simulink model "rx2"  (R2022b)
settings: Solver=FixedStepDiscrete  StartTime=0.0  StopTime=3.3E6  FixedStep=1  RelTol=1e-3  EnableMultiTasking=on
model workspace (MAT data in the model file):
  mwTaskManagerKernelLatency = 0
undefined symbols (not defined in the file or in its folder): Add, jsin, magnitude, rom_pilot_conj_tt, Shift
libraries: hdlsllib x3231, whdlutilities x525, simulink x260, whdlmod x112, whdledac x26, dsphdlmathfun2 x24, commchan3 x1
(part 1 of 59)
settings Model: SimulationMode=accelerator  Creator=admin  LastModifiedBy=yangyifei
settings SolverCC: PositivePriorityOrder=on
settings DataIOCC: ExternalInput=data_rx_tt,start_rx_tt,end_rx_tt,valid_rx_tt  LoadExternalInput=on
settings OptimizationCC: DefaultParameterBehavior=Inlined  EnhancedBackFolding=on  PassReuseOutputArgsAs=Individual arguments  ZeroExternalMemoryAtStartup=off  ZeroInternalMemoryAtStartup=off  InitFltsAndDblsToZero=on  MaxStackSize=64  AccelVerboseBuild=on  OptimizeBlockOrder=speed  DifferentSizesBufferReuse=on  OptimizationCustomize=off  EfficientTunableParamExpr=on
settings DebuggingCC: MultiTaskDSMMsg=warning  ParameterTunabilityLossMsg=error
settings HardwareCC: ProdBitPerPointer=32  ProdBitPerSizeT=32  ProdBitPerPtrDiffT=32  ProdLargestAtomicInteger=Long  ProdLargestAtomicFloat=Double  ProdWordSize=32  ProdLongLongMode=on  ProdHWDeviceType=ARM Compatible->ARM Cortex  TargetLongLongMode=on  HardwareBoardFeatureSet=SoCBlockset
settings ModelReferenceCC: EnableRefExpFcnMdlSchedulingChecks=on  ModelReferenceNumInstancesAllowed=Single
settings SFSimCC: MATLABDynamicMemAlloc=off  SimDLAutoTuning=off
settings RTWCC: Description=Embedded Coder  SystemTargetFile=ert.tlc  GenCodeOnly=on  TemplateMakefile=ert_default_tmf  Toolchain=LCC-win64 v2.4.1 | gmake (64-bit Windows)
settings CodeAppCC: ForceParamTrailComments=on  IgnoreCustomStorageClasses=off  OperatorAnnotations=on  SimulinkDataObjDesc=on  SFDataObjDesc=on  InsertBlockDesc=on
settings ERTTargetCC: TargetLangStandard=C99 (ISO)  InlinedParameterPlacement=NonHierarchical  RootIOFormat=Structure reference  ERTCustomFileTemplate=example_file_process.tlc

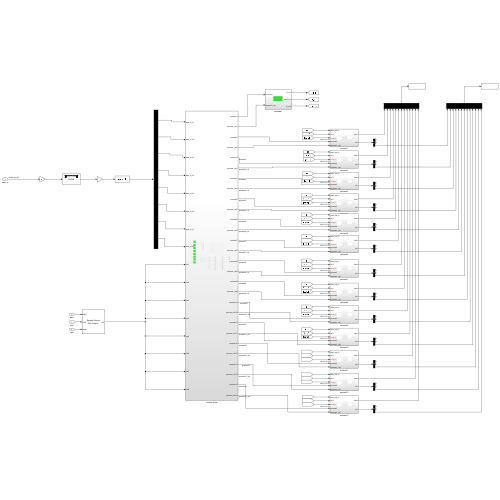
[thumbnail: Simulink's stored preview of the top-level diagram]
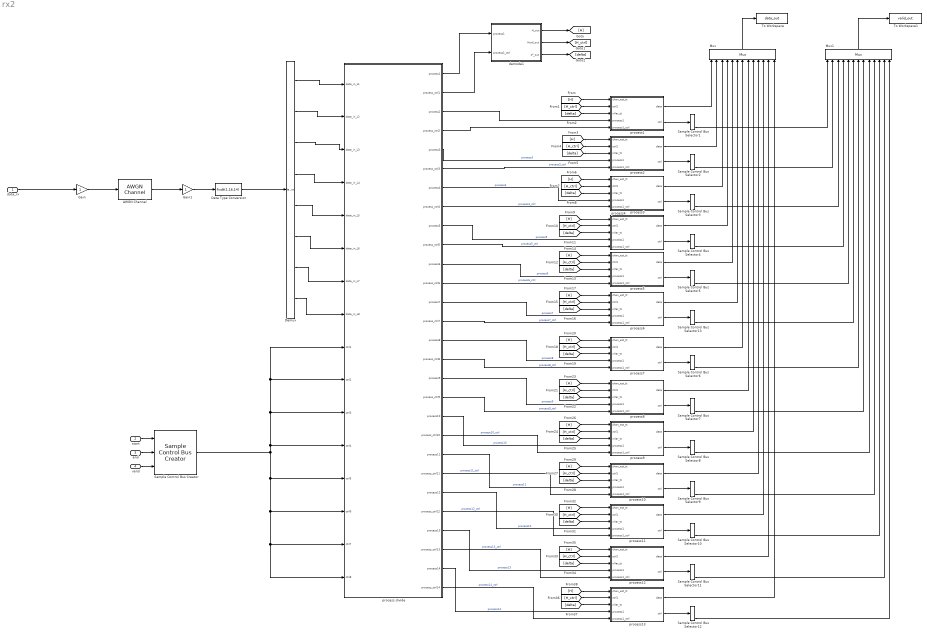
== system rx2 ==
  data_rx : Inport  OutDataTypeStr=double  PortDimensions=8
      settings: SignalType=complex
  start : Inport  Port=2
  end : Inport  Port=3
  valid : Inport  Port=4
  AWGN Channel : commchan3/AWGN Channel  InputProcessing=Columns as channels (frame based)  seed=67  noiseMode="Signal to noise ratio  (SNR)"  EbNodB=10  EsNodB=10  SNRdB=snr  bitsPerSym=1  Ps=1  Tsym=1  variance=1
  Data Type Conversion : DataTypeConversion  OutDataTypeStr=fixdt(1,16,14)  SaturateOnIntegerOverflow=off  RndMeth=Floor
  Demux : Demux  Outputs=8
  Gain : Gain
  Gain1 : Gain
  Mux : Mux  Inputs=13
  Mux1 : Mux  Inputs=13
  Sample Control Bus Creator : whdlutilities/Sample Control Bus Creator
  Sample Control Bus Selector{1..13} (13 alike) : whdlutilities/Sample Control Bus Selector  OutputSignals=start,end,valid
  To Workspace : ToWorkspace  VariableName=data_out  SaveFormat=Timeseries  SampleTime=-1
  To Workspace1 : ToWorkspace  VariableName=valid_out  SaveFormat=Timeseries  SampleTime=-1
  demode1 : Subsystem
  process divide : Subsystem
  process1 : Subsystem
  process10 : Subsystem
  process11 : Subsystem
  process12 : Subsystem
  process13 : Subsystem
  process2 : Subsystem
  process3 : Subsystem
  process4 : Subsystem
  process5 : Subsystem
  process6 : Subsystem
  process7 : Subsystem
  process8 : Subsystem
  process9 : Subsystem
  wires:
  process divide/20(process_ctrl10) -> process9/5(process1_ctrl)  "process10_ctrl"
  Demux/3 -> process divide/3(data_in_L3)
  process divide/13(process7) -> process6/4(process1)  "process7"
  process divide/18(process_ctrl9) -> process8/5(process1_ctrl)  "process9_ctrl"
  Demux/1 -> process divide/1(data_in_L1)
  process divide/14(process_ctrl7) -> process6/5(process1_ctrl)  "process7_ctrl"
  process divide/15(process8) -> process7/4(process1)  "process8"
  Demux/7 -> process divide/7(data_in_L7)
  process divide/8(process_ctrl4) -> process3/5(process1_ctrl)  "process4_ctrl"
  process divide/11(process6) -> process5/4(process1)  "process6"
  process divide/5(process3) -> process2/4(process1)  "process3"
  process divide/7(process4) -> process3/4(process1)  "process4"
  process divide/10(process_ctrl5) -> process4/5(process1_ctrl)  "process5_ctrl"
  process divide/9(process5) -> process4/4(process1)  "process5"
  process divide/3(process2) -> process1/4(process1)
  process divide/6(process_ctrl3) -> process2/5(process1_ctrl)  "process3_ctrl"
  [delta] -> process10/3(nVar_tt)
  [H] -> process9/1(chan_est_tt)
  [delta] -> process13/3(nVar_tt)
  [H_ctrl] -> process2/2(ctrl1)
  [delta] -> process11/3(nVar_tt)
  [H_ctrl] -> process11/2(ctrl1)
  process divide/26(process_ctrl13) -> process12/5(process1_ctrl)  "process13_ctrl"
  [H] -> process12/1(chan_est_tt)
  [H_ctrl] -> process10/2(ctrl1)
  process divide/27(process14) -> process13/4(process1)  "process14"
  process divide/17(process9) -> process8/4(process1)  "process9"
  [delta] -> process6/3(nVar_tt)
  process divide/1(process1) -> demode1/1(process1)
  [H] -> process11/1(chan_est_tt)
  [delta] -> process7/3(nVar_tt)
  demode1/2(Hcrtl_out) -> [H_ctrl]
  [H_ctrl] -> process8/2(ctrl1)
  process divide/19(process10) -> process9/4(process1)  "process10"
  Demux/6 -> process divide/6(data_in_L6)
  [H] -> process7/1(chan_est_tt)
  [delta] -> process5/3(nVar_tt)
  [H] -> process13/1(chan_est_tt)
  process divide/23(process12) -> process11/4(process1)  "process12"
  demode1/3(σ²_out) -> [delta]
  [H] -> process6/1(chan_est_tt)
  [H_ctrl] -> process4/2(ctrl1)
  [delta] -> process12/3(nVar_tt)
  [H] -> process8/1(chan_est_tt)
  [H_ctrl] -> process7/2(ctrl1)
  [delta] -> process2/3(nVar_tt)
  [H_ctrl] -> process6/2(ctrl1)
  process divide/22(process_ctrl11) -> process10/5(process1_ctrl)  "process11_ctrl"
  [delta] -> process4/3(nVar_tt)
  [delta] -> process3/3(nVar_tt)
  Demux/2 -> process divide/2("data_in_L2 ")
  [delta] -> process9/3(nVar_tt)
  [delta] -> process8/3(nVar_tt)
  [H_ctrl] -> process3/2(ctrl1)
  process divide/25(process13) -> process12/4(process1)  "process13"
  [H] -> process5/1(chan_est_tt)
  [H] -> process4/1(chan_est_tt)
  [H] -> process10/1(chan_est_tt)
  [H_ctrl] -> process9/2(ctrl1)
  process divide/21(process11) -> process10/4(process1)  "process11"
  process divide/28(process_ctrl14) -> process13/5(process1_ctrl)  "process14_ctrl"
  Demux/5 -> process divide/5(data_in_L5)
  Demux/8 -> process divide/8(data_in_L8)
  [H_ctrl] -> process12/2(ctrl1)
  [delta] -> process1/3(nVar_tt)
  [H_ctrl] -> process13/2(ctrl1)
  [H] -> process1/1(chan_est_tt)
  [H_ctrl] -> process1/2(ctrl1)
  [H] -> process2/1(chan_est_tt)
  [H_ctrl] -> process5/2(ctrl1)
  process divide/16(process_ctrl8) -> process7/5(process1_ctrl)  "process8_ctrl"
  process divide/24(process_ctrl12) -> process11/5(process1_ctrl)  "process12_ctrl"
  process divide/2(process_ctrl1) -> demode1/2(process1_ctrl)
  process divide/12(process_ctrl6) -> process5/5(process1_ctrl)  "process6_ctrl"
  process divide/4(process_ctrl2) -> process1/5(process1_ctrl)
  demode1/1(H_out) -> [H]
  Demux/4 -> process divide/4(data_in_L4)
  [H] -> process3/1(chan_est_tt)
  start/1 -> Sample Control Bus Creator/1
  end/1 -> Sample Control Bus Creator/2
  valid/1 -> Sample Control Bus Creator/3
  Sample Control Bus Creator/1 -> process divide/16(ctrl8), process divide/15(ctrl7), process divide/14(ctrl6), process divide/13(ctrl5), process divide/12(ctrl4), process divide/11(ctrl3), process divide/10(ctrl2), process divide/9(ctrl1)
  process1/1(data) -> Mux/1
  process2/1(data) -> Mux/2
  process3/1(data) -> Mux/3
  process4/1(data) -> Mux/4
  process5/1(data) -> Mux/5
  process6/1(data) -> Mux/6
  process7/1(data) -> Mux/7
  process8/1(data) -> Mux/8
  process9/1(data) -> Mux/9
  process10/1(data) -> Mux/10
  process11/1(data) -> Mux/11
  process13/1(data) -> Mux/13
  process12/1(data) -> Mux/12
  Mux/1 -> To Workspace/1
  process1/2(ctrl) -> Sample Control Bus Selector1/1
  process2/2(ctrl) -> Sample Control Bus Selector2/1
  process3/2(ctrl) -> Sample Control Bus Selector3/1
  process4/2(ctrl) -> Sample Control Bus Selector4/1
  process5/2(ctrl) -> Sample Control Bus Selector5/1
  process7/2(ctrl) -> Sample Control Bus Selector6/1
  process8/2(ctrl) -> Sample Control Bus Selector7/1
  process9/2(ctrl) -> Sample Control Bus Selector8/1
  process10/2(ctrl) -> Sample Control Bus Selector9/1
  process11/2(ctrl) -> Sample Control Bus Selector10/1
  process12/2(ctrl) -> Sample Control Bus Selector11/1
  process13/2(ctrl) -> Sample Control Bus Selector12/1
  process6/2(ctrl) -> Sample Control Bus Selector13/1
  Mux1/1 -> To Workspace1/1
  Sample Control Bus Selector1/3 -> Mux1/1
  Sample Control Bus Selector2/3 -> Mux1/2
  Sample Control Bus Selector3/3 -> Mux1/3
  Sample Control Bus Selector4/3 -> Mux1/4
  Sample Control Bus Selector5/3 -> Mux1/5
  Sample Control Bus Selector13/3 -> Mux1/6
  Sample Control Bus Selector6/3 -> Mux1/7
  Sample Control Bus Selector7/3 -> Mux1/8
  Sample Control Bus Selector8/3 -> Mux1/9
  Sample Control Bus Selector9/3 -> Mux1/10
  Sample Control Bus Selector10/3 -> Mux1/11
  Sample Control Bus Selector11/3 -> Mux1/12
  Sample Control Bus Selector12/3 -> Mux1/13
  AWGN Channel/1 -> Gain1/1
  Gain/1 -> AWGN Channel/1
  Gain1/1 -> Data Type Conversion/1
  Data Type Conversion/1 -> Demux/1
  data_rx/1 -> Gain/1

== system rx2/demode1 ==
  process1 : Inport
  process1_ctrl : Inport  Port=2  OutDataTypeStr=Bus: BUSOFDM1
  chan_est1 : Subsystem
  H_out : Outport
  Hcrtl_out : Outport  Port=2  OutDataTypeStr=Bus: BUSOFDM1
  σ²_out : Outport  Port=3
  wires:
  chan_est1/3(σ²_out) -> σ²_out/1
  chan_est1/2(Hcrtl_out) -> Hcrtl_out/1
  process1/1 -> chan_est1/1(data_in)
  chan_est1/1(H_out) -> H_out/1
  process1_ctrl/1 -> chan_est1/2(ctrl_in)

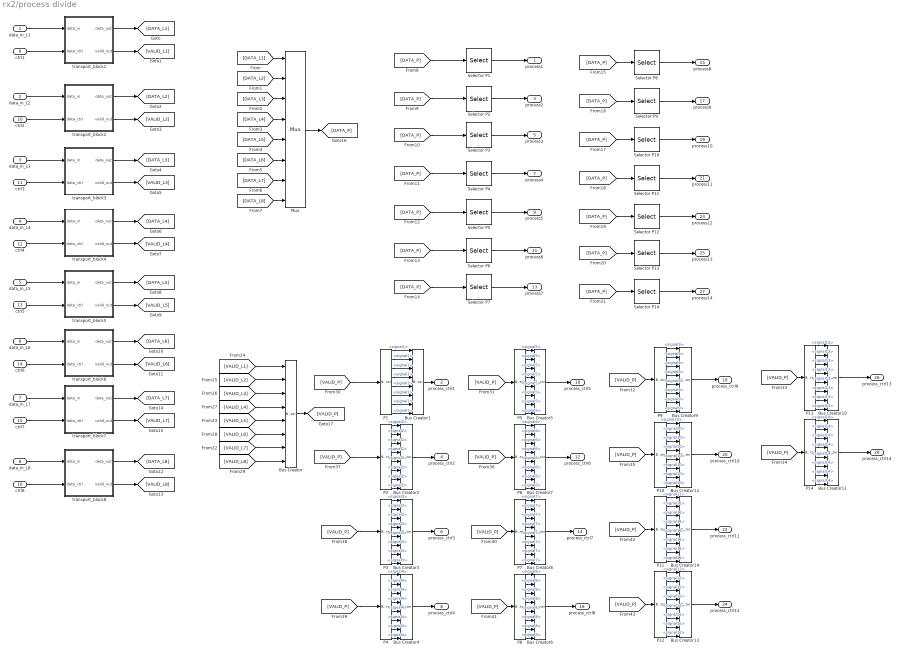
== system rx2/process divide ==
  data_in_L1 : Inport
  "data_in_L2 " : Inport  Port=2
  data_in_L3 : Inport  Port=3
  data_in_L4 : Inport  Port=4
  data_in_L5 : Inport  Port=5
  data_in_L6 : Inport  Port=6
  data_in_L7 : Inport  Port=7
  data_in_L8 : Inport  Port=8
  ctrl1 : Inport  Port=9  OutDataTypeStr=Bus: samplecontrol
  ctrl2 : Inport  Port=10  OutDataTypeStr=Bus: samplecontrol
  ctrl3 : Inport  Port=11  OutDataTypeStr=Bus: samplecontrol
  ctrl4 : Inport  Port=12  OutDataTypeStr=Bus: samplecontrol
  ctrl5 : Inport  Port=13  OutDataTypeStr=Bus: samplecontrol
  ctrl6 : Inport  Port=14  OutDataTypeStr=Bus: samplecontrol
  ctrl7 : Inport  Port=15  OutDataTypeStr=Bus: samplecontrol
  ctrl8 : Inport  Port=16  OutDataTypeStr=Bus: samplecontrol
  Bus Creator{,1..14} (15 alike) : BusCreator  Inputs=8
  Mux : Mux  Inputs=8
  P1 : BusSelector  OutputSignals=signal1.signal1,signal2.signal1,signal3.signal1,signal4.signal1,signal5.signal1,signal6.signal1,signal7.signal1,signal8.signal1
  P10 : BusSelector  OutputSignals=signal1.signal10,signal2.signal10,signal3.signal10,signal4.signal10,signal5.signal10,signal6.signal10,signal7.signal10,signal8.signal10
  P11 : BusSelector  OutputSignals=signal1.signal11,signal2.signal11,signal3.signal11,signal4.signal11,signal5.signal11,signal6.signal11,signal7.signal11,signal8.signal11
  P12 : BusSelector  OutputSignals=signal1.signal12,signal2.signal12,signal3.signal12,signal4.signal12,signal5.signal12,signal6.signal12,signal7.signal12,signal8.signal12
  P13 : BusSelector  OutputSignals=signal1.signal13,signal2.signal13,signal3.signal13,signal4.signal13,signal5.signal13,signal6.signal13,signal7.signal13,signal8.signal13
  P14 : BusSelector  OutputSignals=signal1.signal14,signal2.signal14,signal3.signal14,signal4.signal14,signal5.signal14,signal6.signal14,signal7.signal14,signal8.signal14
  P2 : BusSelector  OutputSignals=signal1.signal2,signal2.signal2,signal3.signal2,signal4.signal2,signal5.signal2,signal6.signal2,signal7.signal2,signal8.signal2
  P3 : BusSelector  OutputSignals=signal1.signal3,signal2.signal3,signal3.signal3,signal4.signal3,signal5.signal3,signal6.signal3,signal7.signal3,signal8.signal3
  P4 : BusSelector  OutputSignals=signal1.signal4,signal2.signal4,signal3.signal4,signal4.signal4,signal5.signal4,signal6.signal4,signal7.signal4,signal8.signal4
  P5 : BusSelector  OutputSignals=signal1.signal5,signal2.signal5,signal3.signal5,signal4.signal5,signal5.signal5,signal6.signal5,signal7.signal5,signal8.signal5
  P6 : BusSelector  OutputSignals=signal1.signal6,signal2.signal6,signal3.signal6,signal4.signal6,signal5.signal6,signal6.signal6,signal7.signal6,signal8.signal6
  P7 : BusSelector  OutputSignals=signal1.signal7,signal2.signal7,signal3.signal7,signal4.signal7,signal5.signal7,signal6.signal7,signal7.signal7,signal8.signal7
  P8 : BusSelector  OutputSignals=signal1.signal8,signal2.signal8,signal3.signal8,signal4.signal8,signal5.signal8,signal6.signal8,signal7.signal8,signal8.signal8
  P9 : BusSelector  OutputSignals=signal1.signal9,signal2.signal9,signal3.signal9,signal4.signal9,signal5.signal9,signal6.signal9,signal7.signal9,signal8.signal9
  Selector P1 : Selector  InputPortWidth=8*14  IndexOptions=Index vector (dialog)  Indices=[1 : 14 :8*14]  OutputSizes=1
  Selector P10 : Selector  InputPortWidth=8*14  IndexOptions=Index vector (dialog)  Indices=[10 : 14 : 8*14]  OutputSizes=1
  Selector P11 : Selector  InputPortWidth=8*14  IndexOptions=Index vector (dialog)  Indices=[11 : 14 :8*14]  OutputSizes=1
  Selector P12 : Selector  InputPortWidth=8*14  IndexOptions=Index vector (dialog)  Indices=[12 : 14 : 8*14]  OutputSizes=1
  Selector P13 : Selector  InputPortWidth=8*14  IndexOptions=Index vector (dialog)  Indices=[13 : 14 :8*14]  OutputSizes=1
  Selector P14 : Selector  InputPortWidth=8*14  IndexOptions=Index vector (dialog)  Indices=[14 : 14 : 8*14]  OutputSizes=1
  Selector P2 : Selector  InputPortWidth=8*14  IndexOptions=Index vector (dialog)  Indices=[2 : 14 : 8*14]  OutputSizes=1
  Selector P3 : Selector  InputPortWidth=8*14  IndexOptions=Index vector (dialog)  Indices=[3 : 14 :8*14]  OutputSizes=1
  Selector P4 : Selector  InputPortWidth=8*14  IndexOptions=Index vector (dialog)  Indices=[4 : 14 : 8*14]  OutputSizes=1
  Selector P5 : Selector  InputPortWidth=8*14  IndexOptions=Index vector (dialog)  Indices=[5: 14 :8*14]  OutputSizes=1
  Selector P6 : Selector  InputPortWidth=8*14  IndexOptions=Index vector (dialog)  Indices=[6: 14 : 8*14]  OutputSizes=1
  Selector P7 : Selector  InputPortWidth=8*14  IndexOptions=Index vector (dialog)  Indices=[7: 14 :8*14]  OutputSizes=1
  Selector P8 : Selector  InputPortWidth=8*14  IndexOptions=Index vector (dialog)  Indices=[8 : 14 : 8*14]  OutputSizes=1
  Selector P9 : Selector  InputPortWidth=8*14  IndexOptions=Index vector (dialog)  Indices=[9 : 14 :8*14]  OutputSizes=1
  transport_block1 : Subsystem
  transport_block2 : Subsystem
  transport_block3 : Subsystem
  transport_block4 : Subsystem
  transport_block5 : Subsystem
  transport_block6 : Subsystem
  transport_block7 : Subsystem
  transport_block8 : Subsystem
  process1 : Outport  VectorParamsAs1DForOutWhenUnconnected=off
  process_ctrl1 : Outport  Port=2  OutDataTypeStr=Bus: BUSOFDM1  VectorParamsAs1DForOutWhenUnconnected=off
  process2 : Outport  Port=3  VectorParamsAs1DForOutWhenUnconnected=off
  process_ctrl2 : Outport  Port=4  OutDataTypeStr=Bus: BUSOFDM1  VectorParamsAs1DForOutWhenUnconnected=off
  process3 : Outport  Port=5  VectorParamsAs1DForOutWhenUnconnected=off
  process_ctrl3 : Outport  Port=6  OutDataTypeStr=Bus: BUSOFDM1  VectorParamsAs1DForOutWhenUnconnected=off
  process4 : Outport  Port=7  VectorParamsAs1DForOutWhenUnconnected=off
  process_ctrl4 : Outport  Port=8  OutDataTypeStr=Bus: BUSOFDM1  VectorParamsAs1DForOutWhenUnconnected=off
  process5 : Outport  Port=9  VectorParamsAs1DForOutWhenUnconnected=off
  process_ctrl5 : Outport  Port=10  OutDataTypeStr=Bus: BUSOFDM1  VectorParamsAs1DForOutWhenUnconnected=off
  process6 : Outport  Port=11  VectorParamsAs1DForOutWhenUnconnected=off
  process_ctrl6 : Outport  Port=12  OutDataTypeStr=Bus: BUSOFDM1  VectorParamsAs1DForOutWhenUnconnected=off
  process7 : Outport  Port=13  VectorParamsAs1DForOutWhenUnconnected=off
  process_ctrl7 : Outport  Port=14  OutDataTypeStr=Bus: BUSOFDM1  VectorParamsAs1DForOutWhenUnconnected=off
  process8 : Outport  Port=15  VectorParamsAs1DForOutWhenUnconnected=off
  process_ctrl8 : Outport  Port=16  OutDataTypeStr=Bus: BUSOFDM1  VectorParamsAs1DForOutWhenUnconnected=off
  process9 : Outport  Port=17  VectorParamsAs1DForOutWhenUnconnected=off
  process_ctrl9 : Outport  Port=18  OutDataTypeStr=Bus: BUSOFDM1  VectorParamsAs1DForOutWhenUnconnected=off
  process10 : Outport  Port=19  VectorParamsAs1DForOutWhenUnconnected=off
  process_ctrl10 : Outport  Port=20  OutDataTypeStr=Bus: BUSOFDM1  VectorParamsAs1DForOutWhenUnconnected=off
  process11 : Outport  Port=21  VectorParamsAs1DForOutWhenUnconnected=off
  process_ctrl11 : Outport  Port=22  OutDataTypeStr=Bus: BUSOFDM1  VectorParamsAs1DForOutWhenUnconnected=off
  process12 : Outport  Port=23  VectorParamsAs1DForOutWhenUnconnected=off
  process_ctrl12 : Outport  Port=24  OutDataTypeStr=Bus: BUSOFDM1  VectorParamsAs1DForOutWhenUnconnected=off
  process13 : Outport  Port=25  VectorParamsAs1DForOutWhenUnconnected=off
  process_ctrl13 : Outport  Port=26  OutDataTypeStr=Bus: BUSOFDM1  VectorParamsAs1DForOutWhenUnconnected=off
  process14 : Outport  Port=27  VectorParamsAs1DForOutWhenUnconnected=off
  process_ctrl14 : Outport  Port=28  OutDataTypeStr=Bus: BUSOFDM1  VectorParamsAs1DForOutWhenUnconnected=off
  wires:
  ctrl1/1 -> transport_block1/2(data_ctrl)
  data_in_L1/1 -> transport_block1/1(data_in)
  "data_in_L2 "/1 -> transport_block2/1(data_in)
  ctrl2/1 -> transport_block2/2(data_ctrl)
  data_in_L3/1 -> transport_block3/1(data_in)
  ctrl3/1 -> transport_block3/2(data_ctrl)
  data_in_L4/1 -> transport_block4/1(data_in)
  ctrl4/1 -> transport_block4/2(data_ctrl)
  data_in_L5/1 -> transport_block5/1(data_in)
  ctrl5/1 -> transport_block5/2(data_ctrl)
  data_in_L6/1 -> transport_block6/1(data_in)
  ctrl6/1 -> transport_block6/2(data_ctrl)
  data_in_L7/1 -> transport_block7/1(data_in)
  ctrl7/1 -> transport_block7/2(data_ctrl)
  data_in_L8/1 -> transport_block8/1(data_in)
  ctrl8/1 -> transport_block8/2(data_ctrl)
  transport_block1/1(data_out) -> [DATA_L1]
  transport_block1/2(valid_out) -> [VALID_L1]
  transport_block2/1(data_out) -> [DATA_L2]
  transport_block2/2(valid_out) -> [VALID_L2]
  transport_block3/1(data_out) -> [DATA_L3]
  transport_block3/2(valid_out) -> [VALID_L3]
  transport_block4/1(data_out) -> [DATA_L4]
  transport_block4/2(valid_out) -> [VALID_L4]
  transport_block5/1(data_out) -> [DATA_L5]
  transport_block5/2(valid_out) -> [VALID_L5]
  transport_block6/1(data_out) -> [DATA_L6]
  transport_block6/2(valid_out) -> [VALID_L6]
  transport_block7/1(data_out) -> [DATA_L7]
  transport_block7/2(valid_out) -> [VALID_L7]
  transport_block8/1(data_out) -> [DATA_L8]
  transport_block8/2(valid_out) -> [VALID_L8]
  [DATA_L1] -> Mux/1
  [DATA_L2] -> Mux/2
  [DATA_L3] -> Mux/3
  [DATA_L4] -> Mux/4
  [DATA_L5] -> Mux/5
  [DATA_L6] -> Mux/6
  [DATA_L8] -> Mux/8
  [DATA_L7] -> Mux/7
  Mux/1 -> [DATA_P]
  [DATA_P] -> Selector P1/1
  [DATA_P] -> Selector P2/1
  [DATA_P] -> Selector P3/1
  [DATA_P] -> Selector P4/1
  [DATA_P] -> Selector P5/1
  [DATA_P] -> Selector P6/1
  [DATA_P] -> Selector P7/1
  [DATA_P] -> Selector P8/1
  [DATA_P] -> Selector P9/1
  [DATA_P] -> Selector P10/1
  [DATA_P] -> Selector P11/1
  [DATA_P] -> Selector P12/1
  [DATA_P] -> Selector P13/1
  [DATA_P] -> Selector P14/1
  [VALID_L7] -> Bus Creator/7
  [VALID_L5] -> Bus Creator/5
  [VALID_L4] -> Bus Creator/4
  [VALID_L3] -> Bus Creator/3
  [VALID_L2] -> Bus Creator/2
  [VALID_L1] -> Bus Creator/1
  [VALID_L6] -> Bus Creator/6
  [VALID_L8] -> Bus Creator/8
  Bus Creator/1 -> [VALID_P]
  [VALID_P] -> P1/1
  [VALID_P] -> P9/1
  [VALID_P] -> P13/1
  [VALID_P] -> P10/1
  [VALID_P] -> P6/1
  [VALID_P] -> P5/1
  [VALID_P] -> P2/1
  [VALID_P] -> P3/1
  [VALID_P] -> P4/1
  [VALID_P] -> P7/1
  [VALID_P] -> P8/1
  [VALID_P] -> P11/1
  [VALID_P] -> P12/1
  [VALID_P] -> P14/1
  P1/1 -> Bus Creator1/1  "<signal1>"
  P1/2 -> Bus Creator1/2  "<signal1>"
  P1/3 -> Bus Creator1/3  "<signal1>"
  P1/4 -> Bus Creator1/4  "<signal1>"
  P1/5 -> Bus Creator1/5  "<signal1>"
  P1/6 -> Bus Creator1/6  "<signal1>"
  P1/7 -> Bus Creator1/7  "<signal1>"
  P1/8 -> Bus Creator1/8  "<signal1>"
  P2/1 -> Bus Creator2/1  "<signal2>"
  P2/2 -> Bus Creator2/2  "<signal2>"
  P2/3 -> Bus Creator2/3  "<signal2>"
  P2/4 -> Bus Creator2/4  "<signal2>"
  P2/5 -> Bus Creator2/5  "<signal2>"
  P2/6 -> Bus Creator2/6  "<signal2>"
  P2/7 -> Bus Creator2/7  "<signal2>"
  P2/8 -> Bus Creator2/8  "<signal2>"
  P3/1 -> Bus Creator3/1  "<signal3>"
  P3/2 -> Bus Creator3/2  "<signal3>"
  P3/3 -> Bus Creator3/3  "<signal3>"
  P3/4 -> Bus Creator3/4  "<signal3>"
  P3/5 -> Bus Creator3/5  "<signal3>"
  P3/6 -> Bus Creator3/6  "<signal3>"
  P3/7 -> Bus Creator3/7  "<signal3>"
  P3/8 -> Bus Creator3/8  "<signal3>"
  P4/1 -> Bus Creator4/1  "<signal4>"
  P4/2 -> Bus Creator4/2  "<signal4>"
  P4/3 -> Bus Creator4/3  "<signal4>"
  P4/4 -> Bus Creator4/4  "<signal4>"
  P4/5 -> Bus Creator4/5  "<signal4>"
  P4/6 -> Bus Creator4/6  "<signal4>"
  P4/7 -> Bus Creator4/7  "<signal4>"
  P4/8 -> Bus Creator4/8  "<signal4>"
  P5/1 -> Bus Creator5/1  "<signal5>"
  P5/2 -> Bus Creator5/2  "<signal5>"
  P5/3 -> Bus Creator5/3  "<signal5>"
  P5/4 -> Bus Creator5/4  "<signal5>"
  P5/5 -> Bus Creator5/5  "<signal5>"
  P5/6 -> Bus Creator5/6  "<signal5>"
  P5/7 -> Bus Creator5/7  "<signal5>"
  P5/8 -> Bus Creator5/8  "<signal5>"
  P8/1 -> Bus Creator6/1  "<signal8>"
  P8/2 -> Bus Creator6/2  "<signal8>"
  P8/3 -> Bus Creator6/3  "<signal8>"
  P8/4 -> Bus Creator6/4  "<signal8>"
  P8/5 -> Bus Creator6/5  "<signal8>"
  P8/6 -> Bus Creator6/6  "<signal8>"
  P8/7 -> Bus Creator6/7  "<signal8>"
  P8/8 -> Bus Creator6/8  "<signal8>"
  P6/1 -> Bus Creator7/1  "<signal6>"
  P6/2 -> Bus Creator7/2  "<signal6>"
  P6/3 -> Bus Creator7/3  "<signal6>"
  P6/4 -> Bus Creator7/4  "<signal6>"
  P6/5 -> Bus Creator7/5  "<signal6>"
  P6/6 -> Bus Creator7/6  "<signal6>"
  P6/7 -> Bus Creator7/7  "<signal6>"
  P6/8 -> Bus Creator7/8  "<signal6>"
  P7/8 -> Bus Creator8/8  "<signal7>"
  P7/7 -> Bus Creator8/7  "<signal7>"
  P7/6 -> Bus Creator8/6  "<signal7>"
  P7/5 -> Bus Creator8/5  "<signal7>"
  P7/4 -> Bus Creator8/4  "<signal7>"
  P7/3 -> Bus Creator8/3  "<signal7>"
  P7/2 -> Bus Creator8/2  "<signal7>"
  P7/1 -> Bus Creator8/1  "<signal7>"
  P9/1 -> Bus Creator9/1  "<signal9>"
  P9/2 -> Bus Creator9/2  "<signal9>"
  P9/3 -> Bus Creator9/3  "<signal9>"
  P9/4 -> Bus Creator9/4  "<signal9>"
  P9/5 -> Bus Creator9/5  "<signal9>"
  P9/6 -> Bus Creator9/6  "<signal9>"
  P9/7 -> Bus Creator9/7  "<signal9>"
  P9/8 -> Bus Creator9/8  "<signal9>"
  P13/1 -> Bus Creator10/1  "<signal13>"
  P13/2 -> Bus Creator10/2  "<signal13>"
  P13/3 -> Bus Creator10/3  "<signal13>"
  P13/4 -> Bus Creator10/4  "<signal13>"
  P13/5 -> Bus Creator10/5  "<signal13>"
  P13/6 -> Bus Creator10/6  "<signal13>"
  P13/7 -> Bus Creator10/7  "<signal13>"
  P13/8 -> Bus Creator10/8  "<signal13>"
  P14/1 -> Bus Creator11/1  "<signal14>"
  P14/2 -> Bus Creator11/2  "<signal14>"
  P14/3 -> Bus Creator11/3  "<signal14>"
  P14/4 -> Bus Creator11/4  "<signal14>"
  P14/5 -> Bus Creator11/5  "<signal14>"
  P14/6 -> Bus Creator11/6  "<signal14>"
  P14/7 -> Bus Creator11/7  "<signal14>"
  P14/8 -> Bus Creator11/8  "<signal14>"
  P10/1 -> Bus Creator12/1  "<signal10>"
  P10/2 -> Bus Creator12/2  "<signal10>"
  P10/3 -> Bus Creator12/3  "<signal10>"
  P10/4 -> Bus Creator12/4  "<signal10>"
  P10/5 -> Bus Creator12/5  "<signal10>"
  P10/6 -> Bus Creator12/6  "<signal10>"
  P10/7 -> Bus Creator12/7  "<signal10>"
  P10/8 -> Bus Creator12/8  "<signal10>"
  P12/1 -> Bus Creator13/1  "<signal12>"
  P12/2 -> Bus Creator13/2  "<signal12>"
  P12/3 -> Bus Creator13/3  "<signal12>"
  P12/4 -> Bus Creator13/4  "<signal12>"
  P12/5 -> Bus Creator13/5  "<signal12>"
  P12/6 -> Bus Creator13/6  "<signal12>"
  P12/7 -> Bus Creator13/7  "<signal12>"
  P12/8 -> Bus Creator13/8  "<signal12>"
  P11/1 -> Bus Creator14/1  "<signal11>"
  P11/2 -> Bus Creator14/2  "<signal11>"
  P11/3 -> Bus Creator14/3  "<signal11>"
  P11/4 -> Bus Creator14/4  "<signal11>"
  P11/5 -> Bus Creator14/5  "<signal11>"
  P11/6 -> Bus Creator14/6  "<signal11>"
  P11/7 -> Bus Creator14/7  "<signal11>"
  P11/8 -> Bus Creator14/8  "<signal11>"
  Selector P1/1 -> process1/1
  Bus Creator1/1 -> process_ctrl1/1
  Selector P2/1 -> process2/1
  Bus Creator2/1 -> process_ctrl2/1
  Selector P3/1 -> process3/1
  Bus Creator3/1 -> process_ctrl3/1
  Selector P4/1 -> process4/1
  Bus Creator4/1 -> process_ctrl4/1
  Selector P5/1 -> process5/1
  Bus Creator5/1 -> process_ctrl5/1
  Selector P6/1 -> process6/1
  Bus Creator7/1 -> process_ctrl6/1
  Selector P7/1 -> process7/1
  Bus Creator8/1 -> process_ctrl7/1
  Selector P8/1 -> process8/1
  Bus Creator6/1 -> process_ctrl8/1
  Selector P9/1 -> process9/1
  Bus Creator9/1 -> process_ctrl9/1
  Selector P10/1 -> process10/1
  Bus Creator12/1 -> process_ctrl10/1
  Selector P11/1 -> process11/1
  Bus Creator14/1 -> process_ctrl11/1
  Selector P12/1 -> process12/1
  Bus Creator13/1 -> process_ctrl12/1
  Selector P13/1 -> process13/1
  Bus Creator10/1 -> process_ctrl13/1
  Selector P14/1 -> process14/1
  Bus Creator11/1 -> process_ctrl14/1

== system rx2/process1 ==
  chan_est_tt : Inport
  ctrl1 : Inport  Port=2  OutDataTypeStr=Bus: BUSOFDM1
  nVar_tt : Inport  Port=3  OutDataTypeStr=fixdt(0,16,12)
  process1 : Inport  Port=4
  process1_ctrl : Inport  Port=5  OutDataTypeStr=Bus: BUSOFDM1
  OFDM_DEMOD1 : Subsystem
  decoder : Subsystem
  data : Outport
  ctrl : Outport  Port=2
  wires:
  process1_ctrl/1 -> OFDM_DEMOD1/2(process_ctrl)
  process1/1 -> OFDM_DEMOD1/1(process)
  ctrl1/1 -> decoder/2(port1_ctrl)
  chan_est_tt/1 -> decoder/1(chan_est_tt1)
  OFDM_DEMOD1/1(rxsig) -> decoder/3(rxSig_tt1)
  OFDM_DEMOD1/2(Rcrtl_out) -> decoder/4(port2_ctrl)
  decoder/1(data_out) -> data/1
  decoder/2(valid_out) -> ctrl/1
  nVar_tt/1 -> decoder/5(nVar_tt)

== system rx2/process10 ==
  chan_est_tt : Inport
  ctrl1 : Inport  Port=2  OutDataTypeStr=Bus: BUSOFDM1
  nVar_tt : Inport  Port=3  OutDataTypeStr=fixdt(0,16,12)
  process1 : Inport  Port=4
  process1_ctrl : Inport  Port=5  OutDataTypeStr=Bus: BUSOFDM1
  OFDM_DEMOD1 : Subsystem
  decoder : Subsystem
  data : Outport
  ctrl : Outport  Port=2
  wires:
  nVar_tt/1 -> decoder/5(nVar_tt)
  decoder/2(valid_out) -> ctrl/1
  decoder/1(data_out) -> data/1
  OFDM_DEMOD1/2(Rcrtl_out) -> decoder/4(port2_ctrl)
  OFDM_DEMOD1/1(rxsig) -> decoder/3(rxSig_tt1)
  chan_est_tt/1 -> decoder/1(chan_est_tt1)
  ctrl1/1 -> decoder/2(port1_ctrl)
  process1/1 -> OFDM_DEMOD1/1(process)
  process1_ctrl/1 -> OFDM_DEMOD1/2(process_ctrl)

== system rx2/process11 ==
  chan_est_tt : Inport
  ctrl1 : Inport  Port=2  OutDataTypeStr=Bus: BUSOFDM1
  nVar_tt : Inport  Port=3  OutDataTypeStr=fixdt(0,16,12)
  process1 : Inport  Port=4
  process1_ctrl : Inport  Port=5  OutDataTypeStr=Bus: BUSOFDM1
  OFDM_DEMOD1 : Subsystem
  decoder : Subsystem
  data : Outport
  ctrl : Outport  Port=2
  wires:
  process1_ctrl/1 -> OFDM_DEMOD1/2(process_ctrl)
  process1/1 -> OFDM_DEMOD1/1(process)
  ctrl1/1 -> decoder/2(port1_ctrl)
  chan_est_tt/1 -> decoder/1(chan_est_tt1)
  OFDM_DEMOD1/1(rxsig) -> decoder/3(rxSig_tt1)
  OFDM_DEMOD1/2(Rcrtl_out) -> decoder/4(port2_ctrl)
  decoder/1(data_out) -> data/1
  decoder/2(valid_out) -> ctrl/1
  nVar_tt/1 -> decoder/5(nVar_tt)

== system rx2/process12 ==
  chan_est_tt : Inport
  ctrl1 : Inport  Port=2  OutDataTypeStr=Bus: BUSOFDM1
  nVar_tt : Inport  Port=3  OutDataTypeStr=fixdt(0,16,12)
  process1 : Inport  Port=4
  process1_ctrl : Inport  Port=5  OutDataTypeStr=Bus: BUSOFDM1
  OFDM_DEMOD1 : Subsystem
  decoder : Subsystem
  data : Outport
  ctrl : Outport  Port=2
  wires:
  nVar_tt/1 -> decoder/5(nVar_tt)
  decoder/2(valid_out) -> ctrl/1
  decoder/1(data_out) -> data/1
  OFDM_DEMOD1/2(Rcrtl_out) -> decoder/4(port2_ctrl)
  OFDM_DEMOD1/1(rxsig) -> decoder/3(rxSig_tt1)
  chan_est_tt/1 -> decoder/1(chan_est_tt1)
  ctrl1/1 -> decoder/2(port1_ctrl)
  process1/1 -> OFDM_DEMOD1/1(process)
  process1_ctrl/1 -> OFDM_DEMOD1/2(process_ctrl)

== system rx2/process13 ==
  chan_est_tt : Inport
  ctrl1 : Inport  Port=2  OutDataTypeStr=Bus: BUSOFDM1
  nVar_tt : Inport  Port=3  OutDataTypeStr=fixdt(0,16,12)
  process1 : Inport  Port=4
  process1_ctrl : Inport  Port=5  OutDataTypeStr=Bus: BUSOFDM1
  OFDM_DEMOD1 : Subsystem
  decoder : Subsystem
  data : Outport
  ctrl : Outport  Port=2
  wires:
  process1_ctrl/1 -> OFDM_DEMOD1/2(process_ctrl)
  process1/1 -> OFDM_DEMOD1/1(process)
  ctrl1/1 -> decoder/2(port1_ctrl)
  chan_est_tt/1 -> decoder/1(chan_est_tt1)
  OFDM_DEMOD1/1(rxsig) -> decoder/3(rxSig_tt1)
  OFDM_DEMOD1/2(Rcrtl_out) -> decoder/4(port2_ctrl)
  decoder/1(data_out) -> data/1
  decoder/2(valid_out) -> ctrl/1
  nVar_tt/1 -> decoder/5(nVar_tt)

== system rx2/process2 ==
  chan_est_tt : Inport
  ctrl1 : Inport  Port=2  OutDataTypeStr=Bus: BUSOFDM1
  nVar_tt : Inport  Port=3  OutDataTypeStr=fixdt(0,16,12)
  process1 : Inport  Port=4
  process1_ctrl : Inport  Port=5  OutDataTypeStr=Bus: BUSOFDM1
  OFDM_DEMOD1 : Subsystem
  decoder : Subsystem
  data : Outport
  ctrl : Outport  Port=2
  wires:
  nVar_tt/1 -> decoder/5(nVar_tt)
  decoder/2(valid_out) -> ctrl/1
  decoder/1(data_out) -> data/1
  OFDM_DEMOD1/2(Rcrtl_out) -> decoder/4(port2_ctrl)
  OFDM_DEMOD1/1(rxsig) -> decoder/3(rxSig_tt1)
  chan_est_tt/1 -> decoder/1(chan_est_tt1)
  ctrl1/1 -> decoder/2(port1_ctrl)
  process1/1 -> OFDM_DEMOD1/1(process)
  process1_ctrl/1 -> OFDM_DEMOD1/2(process_ctrl)

== system rx2/process3 ==
  chan_est_tt : Inport
  ctrl1 : Inport  Port=2  OutDataTypeStr=Bus: BUSOFDM1
  nVar_tt : Inport  Port=3  OutDataTypeStr=fixdt(0,16,12)
  process1 : Inport  Port=4
  process1_ctrl : Inport  Port=5  OutDataTypeStr=Bus: BUSOFDM1
  OFDM_DEMOD1 : Subsystem
  decoder : Subsystem
  data : Outport
  ctrl : Outport  Port=2
  wires:
  process1_ctrl/1 -> OFDM_DEMOD1/2(process_ctrl)
  process1/1 -> OFDM_DEMOD1/1(process)
  ctrl1/1 -> decoder/2(port1_ctrl)
  chan_est_tt/1 -> decoder/1(chan_est_tt1)
  OFDM_DEMOD1/1(rxsig) -> decoder/3(rxSig_tt1)
  OFDM_DEMOD1/2(Rcrtl_out) -> decoder/4(port2_ctrl)
  decoder/1(data_out) -> data/1
  decoder/2(valid_out) -> ctrl/1
  nVar_tt/1 -> decoder/5(nVar_tt)

== system rx2/process4 ==
  chan_est_tt : Inport
  ctrl1 : Inport  Port=2  OutDataTypeStr=Bus: BUSOFDM1
  nVar_tt : Inport  Port=3  OutDataTypeStr=fixdt(0,16,12)
  process1 : Inport  Port=4
  process1_ctrl : Inport  Port=5  OutDataTypeStr=Bus: BUSOFDM1
  OFDM_DEMOD1 : Subsystem
  decoder : Subsystem
  data : Outport
  ctrl : Outport  Port=2
  wires:
  nVar_tt/1 -> decoder/5(nVar_tt)
  decoder/2(valid_out) -> ctrl/1
  decoder/1(data_out) -> data/1
  OFDM_DEMOD1/2(Rcrtl_out) -> decoder/4(port2_ctrl)
  OFDM_DEMOD1/1(rxsig) -> decoder/3(rxSig_tt1)
  chan_est_tt/1 -> decoder/1(chan_est_tt1)
  ctrl1/1 -> decoder/2(port1_ctrl)
  process1/1 -> OFDM_DEMOD1/1(process)
  process1_ctrl/1 -> OFDM_DEMOD1/2(process_ctrl)

== system rx2/process5 ==
  chan_est_tt : Inport
  ctrl1 : Inport  Port=2  OutDataTypeStr=Bus: BUSOFDM1
  nVar_tt : Inport  Port=3  OutDataTypeStr=fixdt(0,16,12)
  process1 : Inport  Port=4
  process1_ctrl : Inport  Port=5  OutDataTypeStr=Bus: BUSOFDM1
  OFDM_DEMOD1 : Subsystem
  decoder : Subsystem
  data : Outport
  ctrl : Outport  Port=2
  wires:
  process1_ctrl/1 -> OFDM_DEMOD1/2(process_ctrl)
  process1/1 -> OFDM_DEMOD1/1(process)
  ctrl1/1 -> decoder/2(port1_ctrl)
  chan_est_tt/1 -> decoder/1(chan_est_tt1)
  OFDM_DEMOD1/1(rxsig) -> decoder/3(rxSig_tt1)
  OFDM_DEMOD1/2(Rcrtl_out) -> decoder/4(port2_ctrl)
  decoder/1(data_out) -> data/1
  decoder/2(valid_out) -> ctrl/1
  nVar_tt/1 -> decoder/5(nVar_tt)

== system rx2/process6 ==
  chan_est_tt : Inport
  ctrl1 : Inport  Port=2  OutDataTypeStr=Bus: BUSOFDM1
  nVar_tt : Inport  Port=3  OutDataTypeStr=fixdt(0,16,12)
  process1 : Inport  Port=4
  process1_ctrl : Inport  Port=5  OutDataTypeStr=Bus: BUSOFDM1
  OFDM_DEMOD1 : Subsystem
  decoder : Subsystem
  data : Outport
  ctrl : Outport  Port=2
  wires:
  nVar_tt/1 -> decoder/5(nVar_tt)
  decoder/2(valid_out) -> ctrl/1
  decoder/1(data_out) -> data/1
  OFDM_DEMOD1/2(Rcrtl_out) -> decoder/4(port2_ctrl)
  OFDM_DEMOD1/1(rxsig) -> decoder/3(rxSig_tt1)
  chan_est_tt/1 -> decoder/1(chan_est_tt1)
  ctrl1/1 -> decoder/2(port1_ctrl)
  process1/1 -> OFDM_DEMOD1/1(process)
  process1_ctrl/1 -> OFDM_DEMOD1/2(process_ctrl)

== system rx2/process7 ==
  chan_est_tt : Inport
  ctrl1 : Inport  Port=2  OutDataTypeStr=Bus: BUSOFDM1
  nVar_tt : Inport  Port=3  OutDataTypeStr=fixdt(0,16,12)
  process1 : Inport  Port=4
  process1_ctrl : Inport  Port=5  OutDataTypeStr=Bus: BUSOFDM1
  OFDM_DEMOD1 : Subsystem
  decoder : Subsystem
  data : Outport
  ctrl : Outport  Port=2
  wires:
  process1_ctrl/1 -> OFDM_DEMOD1/2(process_ctrl)
  process1/1 -> OFDM_DEMOD1/1(process)
  ctrl1/1 -> decoder/2(port1_ctrl)
  chan_est_tt/1 -> decoder/1(chan_est_tt1)
  OFDM_DEMOD1/1(rxsig) -> decoder/3(rxSig_tt1)
  OFDM_DEMOD1/2(Rcrtl_out) -> decoder/4(port2_ctrl)
  decoder/1(data_out) -> data/1
  decoder/2(valid_out) -> ctrl/1
  nVar_tt/1 -> decoder/5(nVar_tt)

== system rx2/process8 ==
  chan_est_tt : Inport
  ctrl1 : Inport  Port=2  OutDataTypeStr=Bus: BUSOFDM1
  nVar_tt : Inport  Port=3  OutDataTypeStr=fixdt(0,16,12)
  process1 : Inport  Port=4
  process1_ctrl : Inport  Port=5  OutDataTypeStr=Bus: BUSOFDM1
  OFDM_DEMOD1 : Subsystem
  decoder : Subsystem
  data : Outport
  ctrl : Outport  Port=2
  wires:
  nVar_tt/1 -> decoder/5(nVar_tt)
  decoder/2(valid_out) -> ctrl/1
  decoder/1(data_out) -> data/1
  OFDM_DEMOD1/2(Rcrtl_out) -> decoder/4(port2_ctrl)
  OFDM_DEMOD1/1(rxsig) -> decoder/3(rxSig_tt1)
  chan_est_tt/1 -> decoder/1(chan_est_tt1)
  ctrl1/1 -> decoder/2(port1_ctrl)
  process1/1 -> OFDM_DEMOD1/1(process)
  process1_ctrl/1 -> OFDM_DEMOD1/2(process_ctrl)

== system rx2/process9 ==
  chan_est_tt : Inport
  ctrl1 : Inport  Port=2  OutDataTypeStr=Bus: BUSOFDM1
  nVar_tt : Inport  Port=3  OutDataTypeStr=fixdt(0,16,12)
  process1 : Inport  Port=4
  process1_ctrl : Inport  Port=5  OutDataTypeStr=Bus: BUSOFDM1
  OFDM_DEMOD1 : Subsystem
  decoder : Subsystem
  data : Outport
  ctrl : Outport  Port=2
  wires:
  process1_ctrl/1 -> OFDM_DEMOD1/2(process_ctrl)
  process1/1 -> OFDM_DEMOD1/1(process)
  ctrl1/1 -> decoder/2(port1_ctrl)
  chan_est_tt/1 -> decoder/1(chan_est_tt1)
  OFDM_DEMOD1/1(rxsig) -> decoder/3(rxSig_tt1)
  OFDM_DEMOD1/2(Rcrtl_out) -> decoder/4(port2_ctrl)
  decoder/1(data_out) -> data/1
  decoder/2(valid_out) -> ctrl/1
  nVar_tt/1 -> decoder/5(nVar_tt)

== system rx2/demode1/chan_est1 ==
  data_in : Inport
  ctrl_in : Inport  Port=2  OutDataTypeStr=Bus: BUSOFDM1
  Subsystem : Subsystem
  H_out : Outport  VectorParamsAs1DForOutWhenUnconnected=off
  Hcrtl_out : Outport  Port=2  OutDataTypeStr=Bus: BUSOFDM1
  σ²_out : Outport  Port=3
  wires:
  data_in/1 -> Subsystem/1(data_in)
  Subsystem/1(H_out) -> H_out/1
  Subsystem/2(crtl_out) -> Hcrtl_out/1
  Subsystem/3(σ²_out) -> σ²_out/1
  ctrl_in/1 -> Subsystem/2(ctrl_in)

== system rx2/process divide/transport_block1 ==
  data_in : Inport
  data_ctrl : Inport  Port=2  OutDataTypeStr=Bus: samplecontrol
  Bus Creator : BusCreator  Inputs=14
  Compare To Constant : hdlsllib/Logic and Bit Operations/Compare To Constant  relop===  const=1  OutDataTypeStr=boolean
  Compare To Constant1 : hdlsllib/Logic and Bit Operations/Compare To Constant  relop===  const=2  OutDataTypeStr=boolean
  Compare To Constant10 : hdlsllib/Logic and Bit Operations/Compare To Constant  relop===  const=11  OutDataTypeStr=boolean
  Compare To Constant11 : hdlsllib/Logic and Bit Operations/Compare To Constant  relop===  const=12  OutDataTypeStr=boolean
  Compare To Constant12 : hdlsllib/Logic and Bit Operations/Compare To Constant  relop===  const=13  OutDataTypeStr=boolean
  Compare To Constant13 : hdlsllib/Logic and Bit Operations/Compare To Constant  relop===  const=14  OutDataTypeStr=boolean
  Compare To Constant2 : hdlsllib/Logic and Bit Operations/Compare To Constant  relop===  const=3  OutDataTypeStr=boolean
  Compare To Constant3 : hdlsllib/Logic and Bit Operations/Compare To Constant  relop===  const=4  OutDataTypeStr=boolean
  Compare To Constant4 : hdlsllib/Logic and Bit Operations/Compare To Constant  relop===  const=5  OutDataTypeStr=boolean
  Compare To Constant5 : hdlsllib/Logic and Bit Operations/Compare To Constant  relop===  const=6  OutDataTypeStr=boolean
  Compare To Constant6 : hdlsllib/Logic and Bit Operations/Compare To Constant  relop===  const=7  OutDataTypeStr=boolean
  Compare To Constant7 : hdlsllib/Logic and Bit Operations/Compare To Constant  relop===  const=8  OutDataTypeStr=boolean
  Compare To Constant8 : hdlsllib/Logic and Bit Operations/Compare To Constant  relop===  const=9  OutDataTypeStr=boolean
  Compare To Constant9 : hdlsllib/Logic and Bit Operations/Compare To Constant  relop===  const=10  OutDataTypeStr=boolean
  Constant : Constant  Value=0  OutDataTypeStr=uint8
  Delay : Delay  DelayLength=1  InitialCondition=0
  Delay1 : Delay  DelayLength=1  InitialCondition=0
  HDL Counter : hdlsllib/Sources/HDL Counter  CountType=Count limited  CountInit=1  CountStep=1  CountMax=14  CountFromType=Initial value  CountFrom=1  CountResetPort=off  CountLoadPort=off  CountEnbPort=on  CountDirPort=off  CountHitOutputPort=off  CountDataType=Unsigned  CountWordLen=8  CountFracLen=0  CountSampTime=1
  Logical Operator : Logic  AllPortsSameDT=off  OutDataTypeStr=boolean
  Mux : Mux  Inputs=14
  Sample Control Bus Selector : whdlutilities/Sample Control Bus Selector  OutputSignals=start,end,valid
  Subsystem1 : Subsystem
  Subsystem10 : Subsystem
  Subsystem11 : Subsystem
  Subsystem12 : Subsystem
  Subsystem13 : Subsystem
  Subsystem14 : Subsystem
  Subsystem2 : Subsystem
  Subsystem3 : Subsystem
  Subsystem4 : Subsystem
  Subsystem5 : Subsystem
  Subsystem6 : Subsystem
  Subsystem7 : Subsystem
  Subsystem8 : Subsystem
  Subsystem9 : Subsystem
  Switch : Switch  Criteria=u2 ~= 0  SaturateOnIntegerOverflow=off  InputSameDT=off
  data_out : Outport  VectorParamsAs1DForOutWhenUnconnected=off
  valid_out : Outport  Port=2  OutDataTypeStr=Bus: RX_BUSOFDM1  VectorParamsAs1DForOutWhenUnconnected=off
  wires:
  data_in/1 -> Delay/1
  HDL Counter/1 -> Switch/1
  Compare To Constant/1 -> Subsystem1/2(select_valid)
  Compare To Constant1/1 -> Subsystem2/2(select_valid)
  Compare To Constant2/1 -> Subsystem3/2(select_valid)
  Compare To Constant3/1 -> Subsystem4/2(select_valid)
  Compare To Constant4/1 -> Subsystem5/2(select_valid)
  Compare To Constant5/1 -> Subsystem6/2(select_valid)
  Compare To Constant6/1 -> Subsystem7/2(select_valid)
  Compare To Constant7/1 -> Subsystem8/2(select_valid)
  Compare To Constant12/1 -> Subsystem13/2(select_valid)
  Compare To Constant11/1 -> Subsystem12/2(select_valid)
  Compare To Constant10/1 -> Subsystem11/2(select_valid)
  Compare To Constant9/1 -> Subsystem10/2(select_valid)
  Compare To Constant8/1 -> Subsystem9/2(select_valid)
  Delay1/1 -> Compare To Constant13/1, Compare To Constant12/1, Compare To Constant11/1, Compare To Constant10/1, Compare To Constant9/1, Compare To Constant8/1, Compare To Constant7/1, Compare To Constant6/1, Compare To Constant5/1, Compare To Constant4/1, Compare To Constant3/1, Compare To Constant2/1, Compare To Constant1/1, Compare To Constant/1
  Delay/1 -> Subsystem2/1(data_in), Subsystem3/1(data_in), Subsystem4/1(data_in), Subsystem5/1(data_in), Subsystem6/1(data_in), Subsystem7/1(data_in), Subsystem8/1(data_in), Subsystem9/1(data_in), Subsystem10/1(data_in), Subsystem11/1(data_in), Subsystem12/1(data_in), Subsystem14/1(data_in), Subsystem13/1(data_in), Subsystem1/1(data_in)
  Compare To Constant13/1 -> Subsystem14/2(select_valid)
  data_ctrl/1 -> Sample Control Bus Selector/1
  Sample Control Bus Selector/3 -> Logical Operator/2, Switch/2
  Switch/1 -> Delay1/1
  Constant/1 -> Switch/3
  Subsystem1/1(data_out) -> Mux/1
  Subsystem2/1(data_out) -> Mux/2
  Subsystem3/1(data_out) -> Mux/3
  Subsystem4/1(data_out) -> Mux/4
  Subsystem5/1(data_out) -> Mux/5
  Subsystem6/1(data_out) -> Mux/6
  Subsystem7/1(data_out) -> Mux/7
  Subsystem8/1(data_out) -> Mux/8
  Subsystem9/1(data_out) -> Mux/9
  Subsystem10/1(data_out) -> Mux/10
  Subsystem11/1(data_out) -> Mux/11
  Subsystem12/1(data_out) -> Mux/12
  Subsystem13/1(data_out) -> Mux/13
  Subsystem14/1(data_out) -> Mux/14
  Subsystem1/2(ctrl_out) -> Bus Creator/1
  Subsystem2/2(ctrl_out) -> Bus Creator/2
  Subsystem3/2(ctrl_out) -> Bus Creator/3
  Subsystem4/2(ctrl_out) -> Bus Creator/4
  Subsystem5/2(ctrl_out) -> Bus Creator/5
  Subsystem6/2(ctrl_out) -> Bus Creator/6
  Subsystem7/2(ctrl_out) -> Bus Creator/7
  Subsystem8/2(ctrl_out) -> Bus Creator/8
  Subsystem9/2(ctrl_out) -> Bus Creator/9
  Subsystem10/2(ctrl_out) -> Bus Creator/10
  Subsystem11/2(ctrl_out) -> Bus Creator/11
  Subsystem12/2(ctrl_out) -> Bus Creator/12
  Subsystem13/2(ctrl_out) -> Bus Creator/13
  Subsystem14/2(ctrl_out) -> Bus Creator/14
  Bus Creator/1 -> valid_out/1
  Mux/1 -> data_out/1
  Sample Control Bus Selector/2 -> Logical Operator/1
  Logical Operator/1 -> HDL Counter/1

== system rx2/process divide/transport_block2 ==
  data_in : Inport
  data_ctrl : Inport  Port=2  OutDataTypeStr=Bus: samplecontrol
  Bus Creator : BusCreator  Inputs=14
  Compare To Constant : hdlsllib/Logic and Bit Operations/Compare To Constant  relop===  const=1  OutDataTypeStr=boolean
  Compare To Constant1 : hdlsllib/Logic and Bit Operations/Compare To Constant  relop===  const=2  OutDataTypeStr=boolean
  Compare To Constant10 : hdlsllib/Logic and Bit Operations/Compare To Constant  relop===  const=11  OutDataTypeStr=boolean
  Compare To Constant11 : hdlsllib/Logic and Bit Operations/Compare To Constant  relop===  const=12  OutDataTypeStr=boolean
  Compare To Constant12 : hdlsllib/Logic and Bit Operations/Compare To Constant  relop===  const=13  OutDataTypeStr=boolean
  Compare To Constant13 : hdlsllib/Logic and Bit Operations/Compare To Constant  relop===  const=14  OutDataTypeStr=boolean
  Compare To Constant2 : hdlsllib/Logic and Bit Operations/Compare To Constant  relop===  const=3  OutDataTypeStr=boolean
  Compare To Constant3 : hdlsllib/Logic and Bit Operations/Compare To Constant  relop===  const=4  OutDataTypeStr=boolean
  Compare To Constant4 : hdlsllib/Logic and Bit Operations/Compare To Constant  relop===  const=5  OutDataTypeStr=boolean
  Compare To Constant5 : hdlsllib/Logic and Bit Operations/Compare To Constant  relop===  const=6  OutDataTypeStr=boolean
  Compare To Constant6 : hdlsllib/Logic and Bit Operations/Compare To Constant  relop===  const=7  OutDataTypeStr=boolean
  Compare To Constant7 : hdlsllib/Logic and Bit Operations/Compare To Constant  relop===  const=8  OutDataTypeStr=boolean
  Compare To Constant8 : hdlsllib/Logic and Bit Operations/Compare To Constant  relop===  const=9  OutDataTypeStr=boolean
  Compare To Constant9 : hdlsllib/Logic and Bit Operations/Compare To Constant  relop===  const=10  OutDataTypeStr=boolean
  Constant : Constant  Value=0  OutDataTypeStr=uint8
  Delay : Delay  DelayLength=1  InitialCondition=0
  Delay1 : Delay  DelayLength=1  InitialCondition=0
  HDL Counter : hdlsllib/Sources/HDL Counter  CountType=Count limited  CountInit=1  CountStep=1  CountMax=14  CountFromType=Initial value  CountFrom=1  CountResetPort=off  CountLoadPort=off  CountEnbPort=on  CountDirPort=off  CountHitOutputPort=off  CountDataType=Unsigned  CountWordLen=8  CountFracLen=0  CountSampTime=1
  Logical Operator : Logic  AllPortsSameDT=off  OutDataTypeStr=boolean
  Mux : Mux  Inputs=14
  Sample Control Bus Selector : whdlutilities/Sample Control Bus Selector  OutputSignals=start,end,valid
  Subsystem1 : Subsystem
  Subsystem10 : Subsystem
  Subsystem11 : Subsystem
  Subsystem12 : Subsystem
  Subsystem13 : Subsystem
  Subsystem14 : Subsystem
  Subsystem2 : Subsystem
  Subsystem3 : Subsystem
  Subsystem4 : Subsystem
  Subsystem5 : Subsystem
  Subsystem6 : Subsystem
  Subsystem7 : Subsystem
  Subsystem8 : Subsystem
  Subsystem9 : Subsystem
  Switch : Switch  Criteria=u2 ~= 0  SaturateOnIntegerOverflow=off  InputSameDT=off
  data_out : Outport  VectorParamsAs1DForOutWhenUnconnected=off
  valid_out : Outport  Port=2  OutDataTypeStr=Bus: RX_BUSOFDM1  VectorParamsAs1DForOutWhenUnconnected=off
  wires:
  Logical Operator/1 -> HDL Counter/1
  Sample Control Bus Selector/2 -> Logical Operator/1
  Mux/1 -> data_out/1
  Bus Creator/1 -> valid_out/1
  Subsystem14/2(ctrl_out) -> Bus Creator/14
  Subsystem13/2(ctrl_out) -> Bus Creator/13
  Subsystem12/2(ctrl_out) -> Bus Creator/12
  Subsystem11/2(ctrl_out) -> Bus Creator/11
  Subsystem10/2(ctrl_out) -> Bus Creator/10
  Subsystem9/2(ctrl_out) -> Bus Creator/9
  Subsystem8/2(ctrl_out) -> Bus Creator/8
  Subsystem7/2(ctrl_out) -> Bus Creator/7
  Subsystem6/2(ctrl_out) -> Bus Creator/6
  Subsystem5/2(ctrl_out) -> Bus Creator/5
  Subsystem4/2(ctrl_out) -> Bus Creator/4
  Subsystem3/2(ctrl_out) -> Bus Creator/3
  Subsystem2/2(ctrl_out) -> Bus Creator/2
  Subsystem1/2(ctrl_out) -> Bus Creator/1
  Subsystem14/1(data_out) -> Mux/14
  Subsystem13/1(data_out) -> Mux/13
  Subsystem12/1(data_out) -> Mux/12
  Subsystem11/1(data_out) -> Mux/11
  Subsystem10/1(data_out) -> Mux/10
  Subsystem9/1(data_out) -> Mux/9
  Subsystem8/1(data_out) -> Mux/8
  Subsystem7/1(data_out) -> Mux/7
  Subsystem6/1(data_out) -> Mux/6
  Subsystem5/1(data_out) -> Mux/5
  Subsystem4/1(data_out) -> Mux/4
  Subsystem3/1(data_out) -> Mux/3
  Subsystem2/1(data_out) -> Mux/2
  Subsystem1/1(data_out) -> Mux/1
  Constant/1 -> Switch/3
  Switch/1 -> Delay1/1
  Sample Control Bus Selector/3 -> Switch/2, Logical Operator/2
  data_ctrl/1 -> Sample Control Bus Selector/1
  Compare To Constant13/1 -> Subsystem14/2(select_valid)
  Delay/1 -> Subsystem1/1(data_in), Subsystem13/1(data_in), Subsystem14/1(data_in), Subsystem12/1(data_in), Subsystem11/1(data_in), Subsystem10/1(data_in), Subsystem9/1(data_in), Subsystem8/1(data_in), Subsystem7/1(data_in), Subsystem6/1(data_in), Subsystem5/1(data_in), Subsystem4/1(data_in), Subsystem3/1(data_in), Subsystem2/1(data_in)
  Delay1/1 -> Compare To Constant/1, Compare To Constant1/1, Compare To Constant2/1, Compare To Constant3/1, Compare To Constant4/1, Compare To Constant5/1, Compare To Constant6/1, Compare To Constant7/1, Compare To Constant8/1, Compare To Constant9/1, Compare To Constant10/1, Compare To Constant11/1, Compare To Constant12/1, Compare To Constant13/1
  Compare To Constant8/1 -> Subsystem9/2(select_valid)
  Compare To Constant9/1 -> Subsystem10/2(select_valid)
  Compare To Constant10/1 -> Subsystem11/2(select_valid)
  Compare To Constant11/1 -> Subsystem12/2(select_valid)
  Compare To Constant12/1 -> Subsystem13/2(select_valid)
  Compare To Constant7/1 -> Subsystem8/2(select_valid)
  Compare To Constant6/1 -> Subsystem7/2(select_valid)
  Compare To Constant5/1 -> Subsystem6/2(select_valid)
  Compare To Constant4/1 -> Subsystem5/2(select_valid)
  Compare To Constant3/1 -> Subsystem4/2(select_valid)
  Compare To Constant2/1 -> Subsystem3/2(select_valid)
  Compare To Constant1/1 -> Subsystem2/2(select_valid)
  Compare To Constant/1 -> Subsystem1/2(select_valid)
  HDL Counter/1 -> Switch/1
  data_in/1 -> Delay/1
